simulink model "untitled"  (Simulink 8.7)
settings: Solver=ode1  StartTime=0.0  StopTime=100  FixedStep=0.01  RelTol=1e-3
settings Model: Creator=kmichalski  LastModifiedBy=km
settings DataIOCC: SignalLoggingSaveFormat=ModelDataLogs
settings OptimizationCC: ExpressionDepthLimit=2147483647
settings DebuggingCC: SolverPrmCheckMsg=warning  FcnCallInpInsideContextMsg=EnableAllAsWarning  StateNameClashWarn=warning

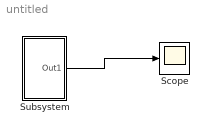
== system untitled ==
  Scope : Scope
  Subsystem : Subsystem  mask{m=10, to=0, l=3, k=1, g=10, fi0=90}
      mask prompts: m "masa"; to "czas odswierzania"; l "dlugosc wahadla"; k "tlumienie"; g "przespieszenie ziemskie"; fi0 "kat wychylenia"
  wires:
  Subsystem/1(Out1) -> Scope/1

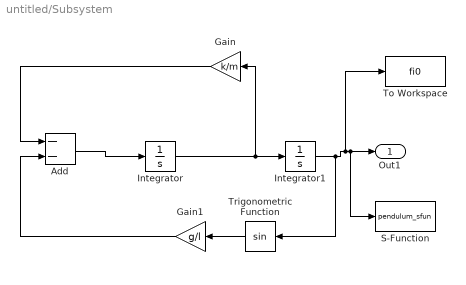
== system untitled/Subsystem ==
  Add : Sum  Inputs=--
  Gain : Gain  Gain=k/m
  Gain1 : Gain  Gain=g/l
  Integrator : Integrator
  Integrator1 : Integrator  InitialCondition=fi0*pi/180
  S-Function : S-Function  FunctionName=pendulum_sfun  Parameters=l,m,fi0,to  SFunctionDeploymentMode=off  EnableBusSupport=off
  To Workspace : ToWorkspace  VariableName=fi0  SampleTime=-1
  Trigonometric Function : Trigonometry
  Out1 : Outport
  wires:
  Trigonometric Function/1 -> Gain1/1
  Integrator1/1 -> Trigonometric Function/1, To Workspace/1, Out1/1, S-Function/1
  Gain1/1 -> Add/2
  Gain/1 -> Add/1
  Integrator/1 -> Integrator1/1, Gain/1
  Add/1 -> Integrator/1
